simulink model "TP25_A47521"  (R2018b)
settings: Solver=ode23tb  StartTime=0.0  StopTime=4*20e-3  RelTol=1e-6
values from neighbouring files (symbols this model uses):
  C1 = 3    [TP25_Dados_A47521.m]
  C2 = 2    [TP25_Dados_A47521.m]
  C3 = 1    [TP25_Dados_A47521.m]
  L1 = 2    [TP25_Dados_A47521.m]
  R1 = 1    [TP25_Dados_A47521.m]
  R2 = 2    [TP25_Dados_A47521.m]
  R3 = 3    [TP25_Dados_A47521.m]
  R4 = 4    [TP25_Dados_A47521.m]
  R5 = 5    [TP25_Dados_A47521.m]
libraries: powerlib x18
settings Model: Creator=Gonçalo  LastModifiedBy=A47521
settings DataIOCC: ReturnWorkspaceOutputs=on

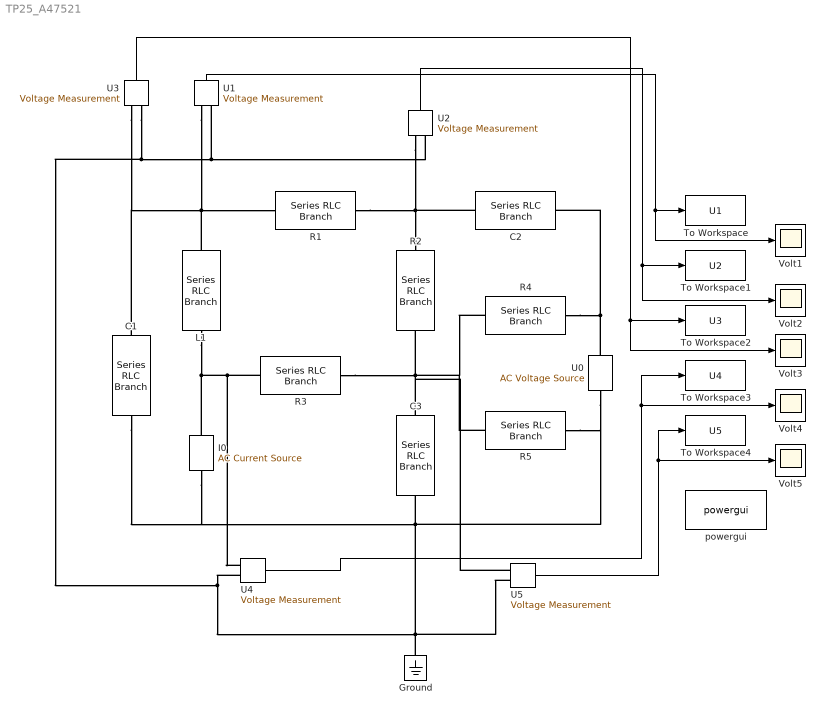
== system TP25_A47521 ==
  C1 : powerlib/Elements/Series RLC Branch  LConnTagsString=__new0  RConnTagsString=__new0  BranchType=C  Resistance=1  Inductance=1e-3  SetiL0=off  InitialCurrent=0  Capacitance=C1  Setx0=off  InitialVoltage=0  Measurements=None
      settings: SourceProductName=Simscape Electrical
  C2 : powerlib/Elements/Series RLC Branch  LConnTagsString=__new0  RConnTagsString=__new0  BranchType=C  Resistance=1  Inductance=1e-3  SetiL0=off  InitialCurrent=0  Capacitance=C2  Setx0=off  InitialVoltage=0  Measurements=None
      settings: SourceProductName=Simscape Electrical
  C3 : powerlib/Elements/Series RLC Branch  LConnTagsString=__new0  RConnTagsString=__new0  BranchType=C  Resistance=R5  Inductance=1e-3  SetiL0=off  InitialCurrent=0  Capacitance=C3  Setx0=off  InitialVoltage=0  Measurements=None
      settings: SourceProductName=Simscape Electrical
  Ground : powerlib/Elements/Ground  LConnTagsString=a
      settings: SourceProductName=Simscape Electrical
  I0 : powerlib/Electrical Sources/AC Current Source  Amplitude=10  Phase=0  Frequency=50  SampleTime=0  Measurements=None
      settings: SourceProductName=Simscape Electrical  SourceProductBaseCode=PS
  L1 : powerlib/Elements/Series RLC Branch  LConnTagsString=__new0  RConnTagsString=__new0  BranchType=L  Resistance=1  Inductance=L1  SetiL0=off  InitialCurrent=0  Capacitance=1e-6  Setx0=off  InitialVoltage=0  Measurements=None
      settings: SourceProductName=Simscape Electrical
  R1 : powerlib/Elements/Series RLC Branch  LConnTagsString=__new0  RConnTagsString=__new0  BranchType=R  Resistance=R1  Inductance=1e-3  SetiL0=off  InitialCurrent=0  Capacitance=1e-6  Setx0=off  InitialVoltage=0  Measurements=None
      settings: SourceProductName=Simscape Electrical
  R2 : powerlib/Elements/Series RLC Branch  LConnTagsString=__new0  RConnTagsString=__new0  BranchType=R  Resistance=R2  Inductance=1e-3  SetiL0=off  InitialCurrent=0  Capacitance=1e-6  Setx0=off  InitialVoltage=0  Measurements=None
      settings: SourceProductName=Simscape Electrical
  R3 : powerlib/Elements/Series RLC Branch  LConnTagsString=__new0  RConnTagsString=__new0  BranchType=R  Resistance=R3  Inductance=1e-3  SetiL0=off  InitialCurrent=0  Capacitance=1e-6  Setx0=off  InitialVoltage=0  Measurements=None
      settings: SourceProductName=Simscape Electrical
  R4 : powerlib/Elements/Series RLC Branch  LConnTagsString=__new0  RConnTagsString=__new0  BranchType=R  Resistance=R4  Inductance=1e-3  SetiL0=off  InitialCurrent=0  Capacitance=1e-6  Setx0=off  InitialVoltage=0  Measurements=None
      settings: SourceProductName=Simscape Electrical
  R5 : powerlib/Elements/Series RLC Branch  LConnTagsString=__new0  RConnTagsString=__new0  BranchType=R  Resistance=R5  Inductance=1e-3  SetiL0=off  InitialCurrent=0  Capacitance=1e-6  Setx0=off  InitialVoltage=0  Measurements=None
      settings: SourceProductName=Simscape Electrical
  To Workspace : ToWorkspace  VariableName=U1  SaveFormat=Timeseries  SampleTime=-1
  To Workspace1 : ToWorkspace  VariableName=U2  SaveFormat=Timeseries  SampleTime=-1
  To Workspace2 : ToWorkspace  VariableName=U3  SaveFormat=Timeseries  SampleTime=-1
  To Workspace3 : ToWorkspace  VariableName=U4  SaveFormat=Timeseries  SampleTime=-1
  To Workspace4 : ToWorkspace  VariableName=U5  SaveFormat=Timeseries  SampleTime=-1
  U0 : powerlib/Electrical Sources/AC Voltage Source  Amplitude=100  Phase=0  Frequency=50  SampleTime=0  Measurements=None  BusType=swing  Pref=10e3  Qref=0  Qmin=-inf  Qmax=+inf
      settings: SourceProductName=Simscape Electrical
  U{1..5} (5 alike) : powerlib/Measurements/Voltage Measurement  PhasorSimulation=off  OutputType=Complex  PSBequivalent=0
      settings: SourceProductName=Simscape Electrical
  Volt{1..5} (5 alike) : Scope
  powergui : powerlib/powergui  Priority=1  SimulationMode=Continuous  SampleTime=50e-6  frequency=60  Iterations=50  frequencyindice=50  Pbase=100e6  ErrMax=1e-4  UnitsV=kV  UnitsW=MW  buscounter=0  FunctionMessages=off  echomessages=off  EnableUseOfTLC=off  CurrentSourceSwitches=off  DisableSnubberDevices=off  DisableRonSwitches=off  DisableVfSwitches=off  DisplayEquations=off  SolverType=Tustin/Backward Euler (TBE)  Interpol=off  ExternalGateDelay=off  methode=off  Ts=100  x0status=blocks  SPID=on  SwTol=0  HookPort=off  RestoreLinks=warning  ResistiveCurrentMeasurement=off  Frange=[0:2:500]  Ylog=off  Xlog=on  ShowGrid=off  save=off  variable=ZData  structure=0  ZoomFFT=off  StartTime=0.0  cycles=1  DisplayStyle=1  fundamental=60  FreqAxis=off  MaxFrequency=1000  frequencyindicesteady=1  RmsSteady=1  display=off
  wires:
  U1/1 -> Volt1/1, To Workspace/1
  U2/1 -> Volt2/1, To Workspace1/1
  U3/1 -> Volt3/1, To Workspace2/1
  U4/1 -> Volt4/1, To Workspace3/1
  U5/1 -> Volt5/1, To Workspace4/1
  connections:
  L1/RConn1 -- C1/LConn1 -- U3/LConn1 -- U1/LConn1 -- R1/LConn1
  R3/LConn1 -- U4/LConn1 -- L1/LConn1 -- I0/RConn1
  C2/LConn1 -- U2/LConn1 -- R1/RConn1 -- R2/LConn1
  R3/RConn1 -- U5/LConn1 -- C3/LConn1 -- R4/RConn1 -- R5/LConn1 -- R2/RConn1
  R4/LConn1 -- U0/RConn1 -- C2/RConn1
  U3/LConn2 -- U2/LConn2 -- U1/LConn2 -- C3/RConn1 -- R5/RConn1 -- U0/LConn1 -- C1/RConn1 -- I0/LConn1 -- U5/LConn2 -- Ground/LConn1 -- U4/LConn2
